simulink model "AEBS_Harness"  (R2022b)
settings: configuration reference "CommonModelConfiguration" (kept outside this file)
undefined symbols (not defined in the file): cc_param_311, cc_param_369, LCFG_ACPE_Timeout, LCFG_AEBS_SignalTimeout
settings Model: Creator=AJOSHI11  LastModifiedBy=AJOSHI11
settings ConfigSetRef: SourceName=CommonModelConfiguration  SourceLocation=Base Workspace

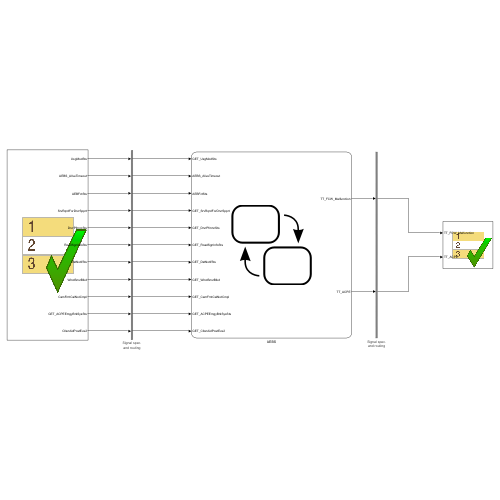
[thumbnail: Simulink's stored preview of the top-level diagram]
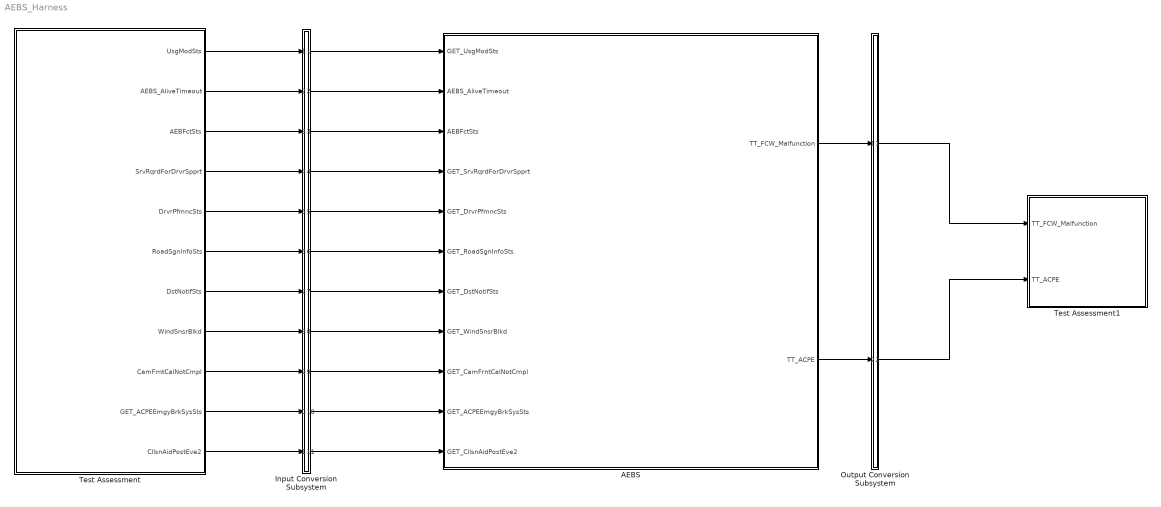
== system AEBS_Harness ==
  AEBS : Stateflow chart  TreatAsAtomicUnit=on
  Input Conversion Subsystem : Subsystem  Tag=__SLT_ICS__  Description=|
      | Signal spec.
      | and routing
      settings: AttributesFormatString=%<Description>
  Output Conversion Subsystem : Subsystem  Tag=__SLT_OCS__  Description=|
      | Signal spec.
      | and routing
      settings: AttributesFormatString=%<Description>
  Test Assessment : Test Sequence  TreatAsAtomicUnit=on
  Test Assessment1 : Test Sequence  TreatAsAtomicUnit=on
  wires:
  Input Conversion Subsystem/1(Outport_1) -> AEBS/1(GET_UsgModSts)
  Input Conversion Subsystem/2(Outport_2) -> AEBS/2(AEBS_AliveTimeout)
  Input Conversion Subsystem/3(Outport_3) -> AEBS/3(AEBFctSts)
  Input Conversion Subsystem/4(Outport_4) -> AEBS/4(GET_SrvRqrdForDrvrSpprt)
  Input Conversion Subsystem/5(Outport_5) -> AEBS/5(GET_DrvrPfmncSts)
  Input Conversion Subsystem/6(Outport_6) -> AEBS/6(GET_RoadSgnInfoSts)
  Input Conversion Subsystem/7(Outport_7) -> AEBS/7(GET_DstNotifSts)
  Input Conversion Subsystem/8(Outport_8) -> AEBS/8(GET_WindSnsrBlkd)
  Input Conversion Subsystem/9(Outport_9) -> AEBS/9(GET_CamFrntCalNotCmpl)
  Input Conversion Subsystem/10(Outport_10) -> AEBS/10(GET_ACPEEmgyBrkSysSts)
  Input Conversion Subsystem/11(Outport_11) -> AEBS/11(GET_CllsnAidPostEve2)
  AEBS/1(TT_FCW_Malfunction) -> Output Conversion Subsystem/1(Inport_1)
  AEBS/2(TT_ACPE) -> Output Conversion Subsystem/2(Inport_2)
  Test Assessment/1(UsgModSts) -> Input Conversion Subsystem/1(Inport_1)
  Test Assessment/2(AEBS_AliveTimeout) -> Input Conversion Subsystem/2(Inport_2)
  Test Assessment/3(AEBFctSts) -> Input Conversion Subsystem/3(Inport_3)
  Test Assessment/4(SrvRqrdForDrvrSpprt) -> Input Conversion Subsystem/4(Inport_4)
  Test Assessment/5(DrvrPfmncSts) -> Input Conversion Subsystem/5(Inport_5)
  Test Assessment/6(RoadSgnInfoSts) -> Input Conversion Subsystem/6(Inport_6)
  Test Assessment/7(DstNotifSts) -> Input Conversion Subsystem/7(Inport_7)
  Test Assessment/8(WindSnsrBlkd) -> Input Conversion Subsystem/8(Inport_8)
  Test Assessment/9(CamFrntCalNotCmpl) -> Input Conversion Subsystem/9(Inport_9)
  Test Assessment/10(GET_ACPEEmgyBrkSysSts) -> Input Conversion Subsystem/10(Inport_10)
  Test Assessment/11(CllsnAidPostEve2) -> Input Conversion Subsystem/11(Inport_11)
  Output Conversion Subsystem/1(Outport_1) -> Test Assessment1/1(TT_FCW_Malfunction)
  Output Conversion Subsystem/2(Outport_2) -> Test Assessment1/2(TT_ACPE)

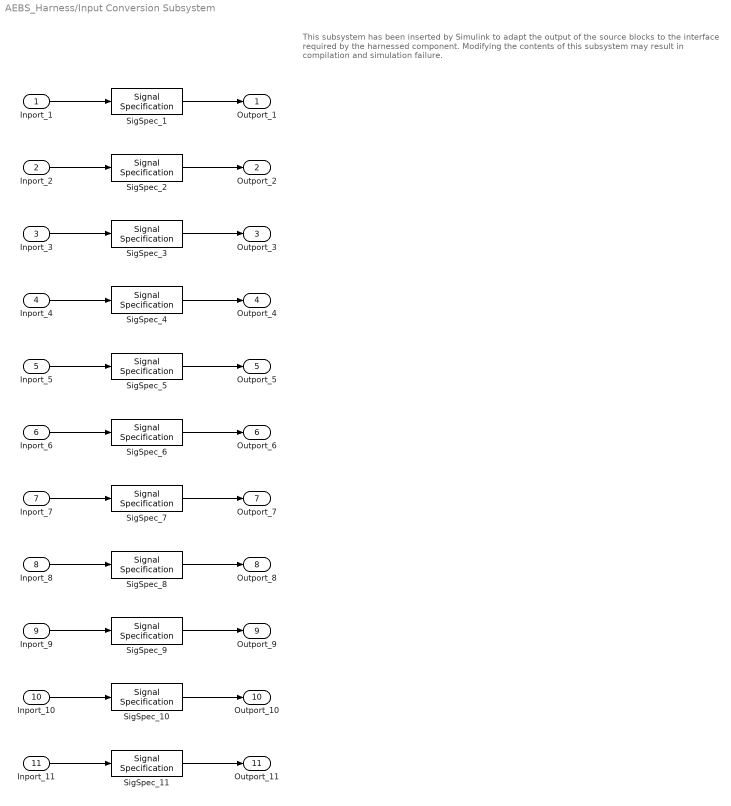
== system AEBS_Harness/Input Conversion Subsystem ==
  note: This subsystem has been inserted by Simulink to adapt the output of the source blocks to the interface required by the harnessed component.
      |  Modifying the contents of this subsystem may result in compilation and simulation failure.
  Inport_1 : Inport
  Inport_2 : Inport  Port=2
  Inport_3 : Inport  Port=3
  Inport_4 : Inport  Port=4
  Inport_5 : Inport  Port=5
  Inport_6 : Inport  Port=6
  Inport_7 : Inport  Port=7
  Inport_8 : Inport  Port=8
  Inport_9 : Inport  Port=9
  Inport_10 : Inport  Port=10
  Inport_11 : Inport  Port=11
  SigSpec_1 : SignalSpecification  OutDataTypeStr=Enum: UsgModSts1  Dimensions=[1]  SampleTime=[0, 0]
  SigSpec_10 : SignalSpecification  OutDataTypeStr=Enum: ACPEEmgyBrkSysSts  Dimensions=[1]  SampleTime=[0, 0]
  SigSpec_11 : SignalSpecification  OutDataTypeStr=Enum: CllsnAidPostEve3  Dimensions=[1]  SampleTime=[0, 0]
  SigSpec_2 : SignalSpecification  OutDataTypeStr=boolean  Dimensions=[1]  SampleTime=[0, 0]
  SigSpec_3 : SignalSpecification  OutDataTypeStr=Enum: UkwnOffOn  Dimensions=[1]  SampleTime=[0, 0]
  SigSpec_4 : SignalSpecification  OutDataTypeStr=Enum: OnOff1  Dimensions=[1]  SampleTime=[0, 0]
  SigSpec_5 : SignalSpecification  OutDataTypeStr=Enum: FctSts2  Dimensions=[1]  SampleTime=[0, 0]
  SigSpec_6 : SignalSpecification  OutDataTypeStr=Enum: FctSts2  Dimensions=[1]  SampleTime=[0, 0]
  SigSpec_7 : SignalSpecification  OutDataTypeStr=Enum: FctSts2  Dimensions=[1]  SampleTime=[0, 0]
  SigSpec_8 : SignalSpecification  OutDataTypeStr=Enum: OnOff1  Dimensions=[1]  SampleTime=[0, 0]
  SigSpec_9 : SignalSpecification  OutDataTypeStr=Enum: NoYes1  Dimensions=[1]  SampleTime=[0, 0]
  Outport_1 : Outport
  Outport_2 : Outport  Port=2
  Outport_3 : Outport  Port=3
  Outport_4 : Outport  Port=4
  Outport_5 : Outport  Port=5
  Outport_6 : Outport  Port=6
  Outport_7 : Outport  Port=7
  Outport_8 : Outport  Port=8
  Outport_9 : Outport  Port=9
  Outport_10 : Outport  Port=10
  Outport_11 : Outport  Port=11
  wires:
  SigSpec_1/1 -> Outport_1/1
  Inport_1/1 -> SigSpec_1/1
  SigSpec_2/1 -> Outport_2/1
  Inport_2/1 -> SigSpec_2/1
  SigSpec_3/1 -> Outport_3/1
  Inport_3/1 -> SigSpec_3/1
  SigSpec_4/1 -> Outport_4/1
  Inport_4/1 -> SigSpec_4/1
  SigSpec_5/1 -> Outport_5/1
  Inport_5/1 -> SigSpec_5/1
  SigSpec_6/1 -> Outport_6/1
  Inport_6/1 -> SigSpec_6/1
  SigSpec_7/1 -> Outport_7/1
  Inport_7/1 -> SigSpec_7/1
  SigSpec_8/1 -> Outport_8/1
  Inport_8/1 -> SigSpec_8/1
  SigSpec_9/1 -> Outport_9/1
  Inport_9/1 -> SigSpec_9/1
  SigSpec_10/1 -> Outport_10/1
  Inport_10/1 -> SigSpec_10/1
  SigSpec_11/1 -> Outport_11/1
  Inport_11/1 -> SigSpec_11/1

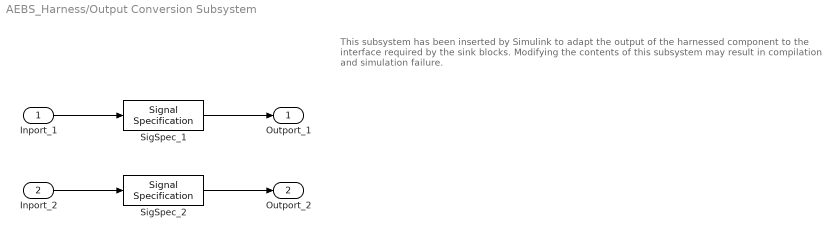
== system AEBS_Harness/Output Conversion Subsystem ==
  note: This subsystem has been inserted by Simulink to adapt the output of the harnessed component to the interface required by the sink blocks.
      |  Modifying the contents of this subsystem may result in compilation and simulation failure.
  Inport_1 : Inport
  Inport_2 : Inport  Port=2
  SigSpec_1 : SignalSpecification  OutDataTypeStr=Bus: PA_StatusAndOffOnChinaValue  Dimensions=[1]  BusOutputAsStruct=on
  SigSpec_2 : SignalSpecification  OutDataTypeStr=Bus: PA_StatusAndOffOnChinaValue  Dimensions=[1]  BusOutputAsStruct=on
  Outport_1 : Outport
  Outport_2 : Outport  Port=2
  wires:
  Inport_1/1 -> SigSpec_1/1
  SigSpec_1/1 -> Outport_1/1
  Inport_2/1 -> SigSpec_2/1
  SigSpec_2/1 -> Outport_2/1

== stateflow chart AEBS_Harness/AEBS ==
  state SYSTEM_OK
    state isActive = activationCheck [function]
      (default) -> (junction 34)
      (junction 34) -> (junction 35) [order 1] : %Engine running
          | [GET_UsgModSts==UsgModSts1.UsgModSts1_UsgModDrvg]
      (junction 34) -> (junction 36) [order 2] : {isActive = false;}
      (junction 35) -> (junction 37) : {isActive = true;}
      (junction 37) -> (junction 36)
      (junction 36) -> (junction 57)
    state NOT_ACTIVE
      entry:
      TT_FCW_Malfunction.Status = E_CommonStatus.Disabled;
      TT_FCW_Malfunction.Value = E_OffOnChina.Off;
      TT_ACPE.Value = E_OffOnChina.Off;
      (default) -> (junction 135)
      (junction 135) -> (junction 136) [order 1] : %Argus3
          | [cc_param_311==3]
      (junction 135) -> (junction 141) [order 2] : %ACPE not present
          | {TT_ACPE.Status =...
          | E_CommonStatus.NotPresent}
      (junction 136) -> (junction 139) : %ACPE present but disabled
          | {TT_ACPE.Status =...
          | E_CommonStatus.Disabled;}
      (junction 139) -> (junction 141)
      (junction 141) -> (junction 146)
    state ACTIVE
      state ACPE [parallel]
        settings: executionOrder=1
        state ACPE_ON
          state ON
            en, du:
            TT_ACPE.Value = E_OffOnChina.On;
          state ON_CHINA
            en, du:
            TT_ACPE.Value = E_OffOnChina.On_China;
          (default) -> (junction 115)
          (junction 115) -> SYSTEM_OK.ACTIVE.ACPE.ACPE_ON.ON [order 2]
          (junction 115) -> (junction 118) [order 1] : %China market
              | [cc_param_369==2]
          (junction 118) -> SYSTEM_OK.ACTIVE.ACPE.ACPE_ON.ON_CHINA
        state ACPE_OFF
          en, du:
          TT_ACPE.Status = E_CommonStatus.Available;
          TT_ACPE.Value = E_OffOnChina.Off;
        state ACPE_NOT_PRESENT
          en, du:
          TT_ACPE.Status = E_CommonStatus.NotPresent;
          TT_ACPE.Value = E_OffOnChina.Off;
        (default) -> (junction 129)
        ACPE_OFF -> ACPE_ON : [hasChangedTo(GET_CllsnAidPostEve2, CllsnAidPostEveArgus3_AcpeFrwd) ||...
            | hasChangedTo(GET_CllsnAidPostEve2, CllsnAidPostEveArgus3_AcpeRrwd)]
        (junction 129) -> ACPE_OFF [order 1] : %Argus3
            | [cc_param_311==3]
        (junction 129) -> (junction 130) [order 2]
        ACPE_ON -> ACPE_OFF : [after(LCFG_ACPE_Timeout, sec)]
        (junction 130) -> ACPE_NOT_PRESENT
      state MALFUNCTION [parallel]
        entry: TT_FCW_Malfunction.Status = E_CommonStatus.Available
        settings: executionOrder=2
        state OFF
          en, du:
          TT_FCW_Malfunction.Value = E_OffOnChina.Off;
        state FAULT_ACTIVE
          state ON
            en, du:
            TT_FCW_Malfunction.Value = E_OffOnChina.On;
          state ON_CHINA
            en, du:
            TT_FCW_Malfunction.Value = E_OffOnChina.On_China;
          (default) -> (junction 94)
          (junction 94) -> SYSTEM_OK.ACTIVE.MALFUNCTION.FAULT_ACTIVE.ON [order 2]
          (junction 94) -> (junction 99) [order 1] : %China market
              | [cc_param_369==2]
          (junction 99) -> SYSTEM_OK.ACTIVE.MALFUNCTION.FAULT_ACTIVE.ON_CHINA
        state ALIVE_TIMEOUT
        (default) -> OFF
        OFF -> FAULT_ACTIVE [order 2] : %AEB function unavailable, telltale activated
            | [AEBFctSts==UkwnOffOn.UkwnOffOn_Off ||...
            | GET_WindSnsrBlkd==OnOff1.OnOff1_On ||...
            | GET_CamFrntCalNotCmpl==NoYes1.NoYes1_Yes ||...
            | GET_DrvrPfmncSts==FctSts2.FctSts2_SrvRqrd ||...
            | GET_DstNotifSts==FctSts2.FctSts2_SrvRqrd ||...
            | GET_RoadSgnInfoSts==FctSts2.FctSts2_SrvRqrd ||...
            | GET_SrvRqrdForDrvrSpprt==OnOff1.OnOff1_On ||...
            | (cc_param_311==3 &&...
            | GET_ACPEEmgyBrkSysSts==ACPEEmgyBrkSysSts_Failure)]
        FAULT_ACTIVE -> OFF : %AEB function available & no AliveTimeout, telltale deactivated
            | [AEBFctSts==UkwnOffOn.UkwnOffOn_On &&...
            | GET_WindSnsrBlkd==OnOff1.OnOff1_Off &&...
            | GET_CamFrntCalNotCmpl==NoYes1.NoYes1_No &&...
            | GET_DrvrPfmncSts~=FctSts2.FctSts2_SrvRqrd &&...
            | GET_DstNotifSts~=FctSts2.FctSts2_SrvRqrd &&...
            | GET_RoadSgnInfoSts~=FctSts2.FctSts2_SrvRqrd &&...
            | GET_SrvRqrdForDrvrSpprt==OnOff1.OnOff1_Off &&...
            | (GET_ACPEEmgyBrkSysSts~=ACPEEmgyBrkSysSts_Failure && cc_param_311==3) &&...
            | AEBS_AliveTimeout==false]
        OFF -> ALIVE_TIMEOUT [order 1] : [AEBS_AliveTimeout==true]
        ALIVE_TIMEOUT -> OFF [order 1] : [AEBS_AliveTimeout==false]
        ALIVE_TIMEOUT -> FAULT_ACTIVE [order 2] : %After LCFG timer has elapsed OR function becomes unavailable
            | [after(LCFG_AEBS_SignalTimeout, sec) || AEBFctSts==OnOff1.OnOff1_Off]
    (default) -> (junction 26)
    (junction 26) -> NOT_ACTIVE [order 1] : [~activationCheck()]
    (junction 26) -> (junction 29) [order 2]
    NOT_ACTIVE -> ACTIVE : [activationCheck()]
    ACTIVE -> NOT_ACTIVE : [~activationCheck()]
    (junction 29) -> ACTIVE
  data: isActive function_output boolean; TT_FCW_Malfunction output Bus: PA_StatusAndOffOnChinaValue; GET_UsgModSts input Enum: UsgModSts1; AEBS_AliveTimeout input boolean; AEBFctSts input Enum: UkwnOffOn; LCFG_AEBS_SignalTimeout parameter uint8; GET_SrvRqrdForDrvrSpprt input Enum: OnOff1; GET_DrvrPfmncSts input Enum: FctSts2; GET_RoadSgnInfoSts input Enum: FctSts2; GET_DstNotifSts input Enum: FctSts2; GET_WindSnsrBlkd input Enum: OnOff1; GET_CamFrntCalNotCmpl input Enum: NoYes1; GET_ACPEEmgyBrkSysSts input; cc_param_369 parameter uint8; GET_CllsnAidPostEve2 input; TT_ACPE output Bus: PA_StatusAndOffOnChinaValue; LCFG_ACPE_Timeout parameter double; cc_param_311 parameter uint8

== stateflow chart AEBS_Harness/Test Assessment ==
  state Initialize_Signals
    UsgModSts = UsgModSts1.UsgModSts1_UsgModAbdnd;
    AEBS_AliveTimeout = false;
    AEBFctSts = UkwnOffOn.UkwnOffOn_Ukwn;
    SrvRqrdForDrvrSpprt = OnOff1.OnOff1_Off;
    DrvrPfmncSts = FctSts2.FctSts2_NotAvl;
    RoadSgnInfoSts = FctSts2.FctSts2_NotAvl;
    DstNotifSts = FctSts2.FctSts2_NotAvl;
    WindSnsrBlkd = OnOff1.OnOff1_Off;
    CamFrntCalNotCmpl = NoYes1.NoYes1_No;
    GET_ACPEEmgyBrkSysSts= ACPEEmgyBrkSysSts.ACPEEmgyBrkSysSts_Failure;
    CllsnAidPostEve2 = CllsnAidPostEve3.CllsnAidPostEve3_NoMsg;
  state TC_AEBS_Status
    state Set_UsageMode_Convinience
      UsgModSts = UsgModSts1.UsgModSts1_UsgModCnvinc;
    (default) -> Set_UsageMode_Convinience
  state Driving_mode
    UsgModSts = UsgModSts1.UsgModSts1_UsgModDrvg;
  state ACPE_ON
    CllsnAidPostEve2 = CllsnAidPostEve3.CllsnAidPostEveArgus3_AcpeFrwd;
  state TC_MALFUNCTION
    AEBFctSts=UkwnOffOn.UkwnOffOn_On;
    WindSnsrBlkd = OnOff1.OnOff1_Off;
    CamFrntCalNotCmpl = NoYes1.NoYes1_No;
    DrvrPfmncSts = FctSts2.FctSts2_Off;
    DstNotifSts = FctSts2.FctSts2_Off;
    RoadSgnInfoSts = FctSts2.FctSts2_Off;
    SrvRqrdForDrvrSpprt = OnOff1.OnOff1_Off;
    GET_ACPEEmgyBrkSysSts = ACPEEmgyBrkSysSts.ACPEEmgyBrkSysSts_NoFailure;
    state ALIVE_TIMEOUT
      AEBS_AliveTimeout = true;
      settings: description=OFF -> ALIVE_TIMEOUT
    state OFF
      AEBS_AliveTimeout = false;
      settings: description=ALIVE_TIMEOUT -> OFF
    state FAULT_ACTIVE_by_ACPE
      GET_ACPEEmgyBrkSysSts= ACPEEmgyBrkSysSts.ACPEEmgyBrkSysSts_Failure;
      settings: description=OFF-> FAULT_ACTIVE
    state OFF1
      GET_ACPEEmgyBrkSysSts= ACPEEmgyBrkSysSts.ACPEEmgyBrkSysSts_NoFailure;
      settings: description=FAULT_ACTIVE->OFF
    state ALIVE_TIMEOUT1
      AEBS_AliveTimeout = true;
      settings: description=OFF->ALIVE_TIMEOUT
    state Set_fctSts_On
      AEBFctSts = UkwnOffOn.UkwnOffOn_On;
      WindSnsrBlkd = OnOff1.OnOff1_Off;
      CamFrntCalNotCmpl = NoYes1.NoYes1_No;
      DrvrPfmncSts = FctSts2.FctSts2_Off;
      DstNotifSts = FctSts2.FctSts2_Off;
      RoadSgnInfoSts = FctSts2.FctSts2_Off;
      SrvRqrdForDrvrSpprt = OnOff1.OnOff1_Off;
      GET_ACPEEmgyBrkSysSts = ACPEEmgyBrkSysSts.ACPEEmgyBrkSysSts_NoFailure;
      AEBS_AliveTimeout = false;
      settings: description=FAULT_ACTIVE->OFF
    (default) -> ALIVE_TIMEOUT
    ALIVE_TIMEOUT -> OFF : [
        | after(2,sec)
        | ]
    OFF -> FAULT_ACTIVE_by_ACPE : [
        | after(2,sec)
        | ]
    FAULT_ACTIVE_by_ACPE -> OFF1 : [
        | after(2,sec)
        | ]
    OFF1 -> ALIVE_TIMEOUT1 : [
        | after(2,sec)
        | ]
    ALIVE_TIMEOUT1 -> Set_fctSts_On : [
        | after(7,sec)
        | ]
  (default) -> Initialize_Signals
  Initialize_Signals -> TC_AEBS_Status
  TC_AEBS_Status -> Driving_mode : [
      | after(2,sec)
      | ]
  Driving_mode -> ACPE_ON : [
      | after(2,sec)
      | ]
  ACPE_ON -> TC_MALFUNCTION : [
      | after(2,sec)
      | ]
  data: UsgModSts output; AEBS_AliveTimeout output; AEBFctSts output; SrvRqrdForDrvrSpprt output; DrvrPfmncSts output; RoadSgnInfoSts output; DstNotifSts output; WindSnsrBlkd output; CamFrntCalNotCmpl output; GET_ACPEEmgyBrkSysSts output; CllsnAidPostEve2 output

== stateflow chart AEBS_Harness/Test Assessment1 ==
  state step_1
    state step_1_1
    state step_1_2
      verify(TT_FCW_Malfunction.Status == E_CommonStatus.Disabled)
      verify(TT_FCW_Malfunction.Value == E_OffOnChina.Off)
      verify(TT_ACPE.Value == E_OffOnChina.Off)
      verify(TT_ACPE.Status == E_CommonStatus.Disabled)
    (default) -> (junction 22)
    step_1 -> (junction 22) [order 1]
    (junction 22) -> (junction 23) [order 1] : [t < 1
        | ]
    (junction 23) -> step_1_1 [order 1] : [~in(step_1.step_1_1)]
    (junction 22) -> (junction 31) [order 2]
    (junction 23) -> (junction 26) [order 2]
    (junction 31) -> (junction 32)
    (junction 32) -> step_1_2 [order 1] : [~in(step_1.step_1_2)]
    (junction 32) -> (junction 35) [order 2]
  state step_2
    verify(TT_ACPE.Status == E_CommonStatus.Available)
    verify(TT_ACPE.Value == E_OffOnChina.Off)
  state step_3
    verify(TT_ACPE.Value == E_OffOnChina.On)
  state step_4
    verify(TT_ACPE.Status == E_CommonStatus.Available)
    verify(TT_ACPE.Value == E_OffOnChina.Off)
    verify(TT_FCW_Malfunction.Status == E_CommonStatus.Available)
    verify(TT_FCW_Malfunction.Value == E_OffOnChina.On)
  state step_5
    verify(TT_FCW_Malfunction.Value == E_OffOnChina.Off)
  state step_6
    verify(TT_FCW_Malfunction.Value == E_OffOnChina.On)
  state step_7
    verify(TT_FCW_Malfunction.Value == E_OffOnChina.Off)
  state step_8
    verify(TT_FCW_Malfunction.Value == E_OffOnChina.On)
  state step_9
    verify(TT_FCW_Malfunction.Value == E_OffOnChina.Off)
  (default) -> step_1
  step_1 -> step_2 [order 1] : [
      | after(2.1,sec)
      | ]
  step_2 -> step_3 : [
      | after(2,sec)
      | ]
  step_3 -> step_4 : [
      | after(2,sec)
      | ]
  step_4 -> step_5 : [
      | after(2,sec)
      | ]
  step_5 -> step_6 : [
      | after(2,sec)
      | ]
  step_6 -> step_7 : [
      | after(2,sec)
      | ]
  step_7 -> step_8 : [
      | after(5.1,sec)
      | ]
  step_8 -> step_9 : [
      | after(2,sec)
      | ]
  data: TT_FCW_Malfunction input; TT_ACPE input
